simulink model "EM21"  (R2024a)
settings: Solver=VariableStepAuto  StartTime=0.0  StopTime=10.0  RelTol=1e-3
libraries: spsThreePhaseVIMeasurementLib x6, spsThreePhaseTransformerTwoWindingsLib x5, spsThreePhaseParallelRLCBranchLib x3, spsThreePhaseSourceLib x3, spsThreePhaseBreakerLib x3, sps_lib x1
settings Model: Creator=ASUS  LastModifiedBy=ASUS

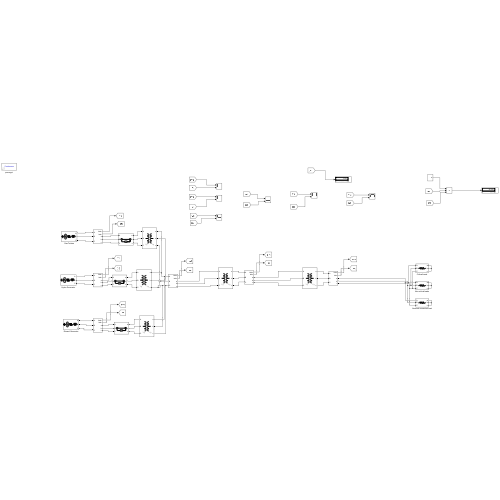
[thumbnail: Simulink's stored preview of the top-level diagram]
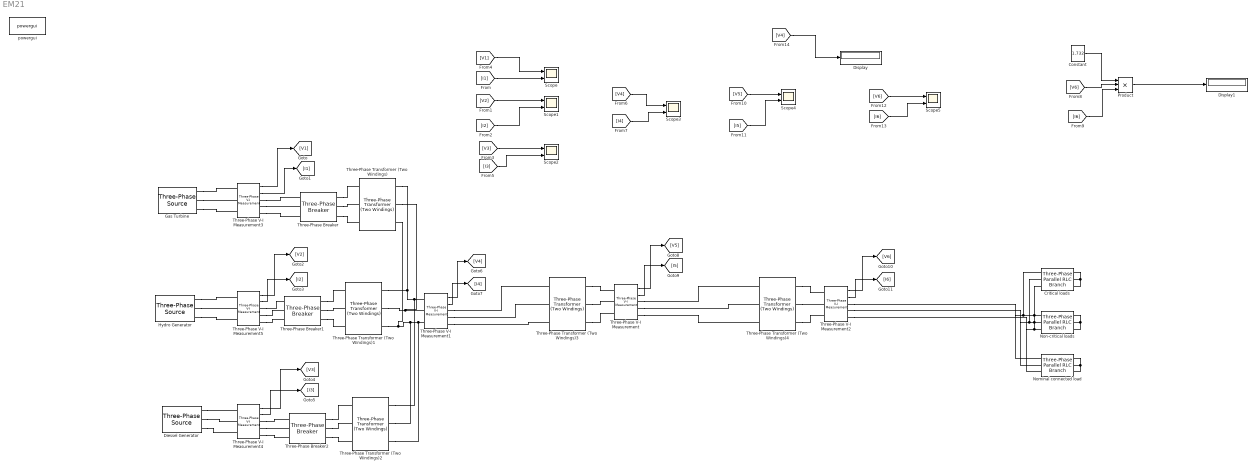
== system EM21 ==
  Constant : Constant  Value=1.732
  Critical loads : spsThreePhaseParallelRLCBranchLib/Three-Phase Parallel RLC Branch  LConnTagsString=A|B|C  RConnTagsString=A|B|C  BranchType=R  Resistance=1000  Inductance=1e-3  Capacitance=1e-6  Measurements=None
  Diessel Generator : spsThreePhaseSourceLib/Three-Phase Source  InternalConnection=Yg  VoltagePhases=off  Voltage=10e3  PhaseAngle=0  Voltage_phases=[25e3 25e3 25e3]/sqrt(3)  PhaseAngles_phases=[0 -120 +120]  Frequency=50  NonIdealSource=on  SpecifyImpedance=off  Resistance=0.8929  Inductance=16.58e-3  ShortCircuitLevel=100e6  BaseVoltage=10e3  XRratio=7  BusType=PV  Pref=4e6  Qref=0  Prefabc=[10e3, 10e3, 10e3]  Qrefabc=[0, 0, 0]  Qmin=-inf  Qmax=inf
  Display : Display
  Display1 : Display
  Gas Turbine : spsThreePhaseSourceLib/Three-Phase Source  InternalConnection=Yg  VoltagePhases=off  Voltage=11e3  PhaseAngle=0  Voltage_phases=[25e3 25e3 25e3]/sqrt(3)  PhaseAngles_phases=[0 -120 +120]  Frequency=50  NonIdealSource=on  SpecifyImpedance=off  Resistance=0.8929  Inductance=16.58e-3  ShortCircuitLevel=100e6  BaseVoltage=11e3  XRratio=7  BusType=PV  Pref=1e6  Qref=0  Prefabc=[10e3, 10e3, 10e3]  Qrefabc=[0, 0, 0]  Qmin=-inf  Qmax=inf
  Hydro Generator : spsThreePhaseSourceLib/Three-Phase Source  InternalConnection=Yg  VoltagePhases=off  Voltage=12e3  PhaseAngle=0  Voltage_phases=[25e3 25e3 25e3]/sqrt(3)  PhaseAngles_phases=[0 -120 +120]  Frequency=50  NonIdealSource=on  SpecifyImpedance=off  Resistance=0.8929  Inductance=16.58e-3  ShortCircuitLevel=100e6  BaseVoltage=12e3  XRratio=7  BusType=PV  Pref=2e6  Qref=0  Prefabc=[10e3, 10e3, 10e3]  Qrefabc=[0, 0, 0]  Qmin=-inf  Qmax=inf
  Nominal connected load : spsThreePhaseParallelRLCBranchLib/Three-Phase Parallel RLC Branch  LConnTagsString=A|B|C  RConnTagsString=A|B|C  BranchType=R  Resistance=1000  Inductance=1e-3  Capacitance=1e-6  Measurements=None
  Non-critical loads : spsThreePhaseParallelRLCBranchLib/Three-Phase Parallel RLC Branch  LConnTagsString=A|B|C  RConnTagsString=A|B|C  BranchType=R  Resistance=1000  Inductance=1e-3  Capacitance=1e-6  Measurements=None
  Product : Product  Inputs=3
  Scope{,1..5} (6 alike) : Scope  NumInputPorts=2
  Three-Phase Transformer (Two Windings) : spsThreePhaseTransformerTwoWindingsLib/Three-Phase Transformer (Two Windings)  Winding1Connection=Yg  Winding2Connection=Yg  CoreType=Three single-phase transformers  SetSaturation=off  Hysteresis=off  DataFile='hysteresis'  SetInitialFlux=off  Measurements=None  UNITS=pu  NominalPower=[ 1e6 , 50 ]  Winding1=[ 11e3 , 0.002 , 0.08 ]  Winding2=[ 132e3 , 0.002 , 0.08 ]  Rm=500  Lm=500  L0=2.866  Saturation=[ 0,0 ; 0.0024,1.2 ; 1.0,1.52 ]  InitialFluxes=[1273.5 -1273.5 1114.3]  BreakLoop=off  DiscreteSolver=Trapezoidal iterative  DataType=off  TransfoNumber=1
  Three-Phase Transformer (Two Windings)1 : spsThreePhaseTransformerTwoWindingsLib/Three-Phase Transformer (Two Windings)  Winding1Connection=Yg  Winding2Connection=Yg  CoreType=Three single-phase transformers  SetSaturation=off  Hysteresis=off  DataFile='hysteresis'  SetInitialFlux=off  Measurements=None  UNITS=pu  NominalPower=[ 2e6 , 50 ]  Winding1=[ 12e3 , 0.002 , 0.08 ]  Winding2=[ 132e3 , 0.002 , 0.08 ]  Rm=500  Lm=500  L0=0.5  Saturation=[ 0,0 ; 0.0024,1.2 ; 1.0,1.52 ]  InitialFluxes=[ 0.8 , -0.8 , 0.7 ]  BreakLoop=off  DiscreteSolver=Trapezoidal iterative  DataType=off  TransfoNumber=1
  Three-Phase Transformer (Two Windings)2 : spsThreePhaseTransformerTwoWindingsLib/Three-Phase Transformer (Two Windings)  Winding1Connection=Yg  Winding2Connection=Yg  CoreType=Three single-phase transformers  SetSaturation=off  Hysteresis=off  DataFile='hysteresis'  SetInitialFlux=off  Measurements=None  UNITS=pu  NominalPower=[ 4e6 , 50 ]  Winding1=[ 10e3 , 0.002 , 0.08 ]  Winding2=[ 132e3 , 0.002 , 0.08 ]  Rm=500  Lm=500  L0=0.5  Saturation=[ 0,0 ; 0.0024,1.2 ; 1.0,1.52 ]  InitialFluxes=[ 0.8 , -0.8 , 0.7 ]  BreakLoop=off  DiscreteSolver=Trapezoidal iterative  DataType=off  TransfoNumber=1
  Three-Phase Transformer (Two Windings)3 : spsThreePhaseTransformerTwoWindingsLib/Three-Phase Transformer (Two Windings)  Winding1Connection=Yg  Winding2Connection=Yg  CoreType=Three single-phase transformers  SetSaturation=off  Hysteresis=off  DataFile='hysteresis'  SetInitialFlux=off  Measurements=None  UNITS=pu  NominalPower=[ 7e6 , 50 ]  Winding1=[ 132e3 , 0.002 , 0.08 ]  Winding2=[ 11e3 , 0.002 , 0.08 ]  Rm=500  Lm=500  L0=0.5  Saturation=[ 0,0 ; 0.0024,1.2 ; 1.0,1.52 ]  InitialFluxes=[ 0.8 , -0.8 , 0.7 ]  BreakLoop=off  DiscreteSolver=Trapezoidal iterative  DataType=off  TransfoNumber=1
  Three-Phase Transformer (Two Windings)4 : spsThreePhaseTransformerTwoWindingsLib/Three-Phase Transformer (Two Windings)  Winding1Connection=Yg  Winding2Connection=Yg  CoreType=Three single-phase transformers  SetSaturation=off  Hysteresis=off  DataFile='hysteresis'  SetInitialFlux=off  Measurements=None  UNITS=pu  NominalPower=[ 7e6 , 50 ]  Winding1=[ 11e3 , 0.002 , 0.08 ]  Winding2=[ 400 , 0.002 , 0.08 ]  Rm=500  Lm=500  L0=0.5  Saturation=[ 0,0 ; 0.0024,1.2 ; 1.0,1.52 ]  InitialFluxes=[ 0.8 , -0.8 , 0.7 ]  BreakLoop=off  DiscreteSolver=Trapezoidal iterative  DataType=off  TransfoNumber=1
  Three-Phase V-I Measurement{,1..5} (6 alike) : spsThreePhaseVIMeasurementLib/Three-Phase V-I Measurement  VoltageMeasurement=phase-to-ground  SetLabelV=off  LabelV=Vabc  Vpu=off  VpuLL=off  CurrentMeasurement=yes  SetLabelI=off  LabelI=Iabc  Ipu=off  Pbase=100e6  Vbase=500e3  OutputType=Complex  PhasorSimulation=off  PSBequivalent=0
  Three-Phase Breaker : spsThreePhaseBreakerLib/Three-Phase Breaker  InitialState=closed  SwitchA=on  SwitchB=on  SwitchC=on  SwitchTimes="[1/60  5/60]"  External=off  BreakerResistance=0.01  SnubberResistance=1e6  SnubberCapacitance=inf  Measurements=None
  Three-Phase Breaker1 : spsThreePhaseBreakerLib/Three-Phase Breaker  InitialState=closed  SwitchA=on  SwitchB=on  SwitchC=on  SwitchTimes="[1/60  5/60]"  External=off  BreakerResistance=0.01  SnubberResistance=1e6  SnubberCapacitance=inf  Measurements=None
  Three-Phase Breaker2 : spsThreePhaseBreakerLib/Three-Phase Breaker  InitialState=closed  SwitchA=on  SwitchB=on  SwitchC=on  SwitchTimes="[1/60  5/60]"  External=off  BreakerResistance=0.01  SnubberResistance=1e6  SnubberCapacitance=inf  Measurements=None
  powergui : sps_lib/powergui  Priority=1  SimulationMode=Continuous  SampleTime=50e-6  frequency=60  Iterations=50  frequencyindice=50  Pbase=100e6  ErrMax=1e-4  UnitsV=kV  UnitsW=MW  buscounter=0  FunctionMessages=off  echomessages=off  EnableUseOfTLC=off  CurrentSourceSwitches=off  DisableSnubberDevices=off  DisableRonSwitches=off  DisableVfSwitches=off  DisplayEquations=off  AutomaticDiscreteSolvers=off  SolverType=Tustin/Backward Euler (TBE)  Interpol=off  ExternalGateDelay=off  methode=off  Ts=100  x0status=blocks  SPID=on  SwTol=0  HookPort=off  NonlinearTolerance=1e-4  nMaxIteration=100  ContinueOnMaxIteration=off  RestoreLinks=warning  ResistiveCurrentMeasurement=off  Frange=[0:2:500]  Ylog=off  Xlog=on  ShowGrid=off  save=off  variable=ZData  structure=0  ZoomFFT=off  StartTime=0.0  cycles=1  DisplayStyle=1  fundamental=60  FreqAxis=off  MaxFrequency=1000  frequencyindicesteady=1  RmsSteady=1  display=off
  wires:
  Three-Phase V-I Measurement3/1 -> [V1]
  Three-Phase V-I Measurement3/2 -> [I1]
  Three-Phase V-I Measurement5/1 -> [V2]
  Three-Phase V-I Measurement5/2 -> [I2]
  Three-Phase V-I Measurement4/1 -> [V3]
  Three-Phase V-I Measurement4/2 -> [I3]
  [V1] -> Scope/1
  [I1] -> Scope/2
  [V2] -> Scope1/1
  [I2] -> Scope1/2
  [V3] -> Scope2/1
  [I3] -> Scope2/2
  Three-Phase V-I Measurement1/1 -> [V4]
  Three-Phase V-I Measurement1/2 -> [I4]
  [V4] -> Scope3/1
  [I4] -> Scope3/2
  Three-Phase V-I Measurement/1 -> [V5]
  Three-Phase V-I Measurement/2 -> [I5]
  Three-Phase V-I Measurement2/1 -> [V6]
  Three-Phase V-I Measurement2/2 -> [I6]
  [V5] -> Scope4/1
  [I5] -> Scope4/2
  [V6] -> Scope5/1
  [I6] -> Scope5/2
  [V4] -> Display/1
  Constant/1 -> Product/1
  [V6] -> Product/2
  [I6] -> Product/3
  Product/1 -> Display1/1
  connections:
  Critical loads/RConn1 -- Critical loads/RConn2 -- Critical loads/RConn3
  Non-critical loads/RConn1 -- Non-critical loads/RConn2 -- Non-critical loads/RConn3
  Nominal connected load/RConn1 -- Nominal connected load/RConn2 -- Nominal connected load/RConn3
  Three-Phase Transformer (Two Windings)1/RConn1 -- Three-Phase Transformer (Two Windings)2/RConn1 -- Three-Phase V-I Measurement1/LConn1 -- Three-Phase Transformer (Two Windings)/RConn1
  Three-Phase Transformer (Two Windings)1/RConn2 -- Three-Phase Transformer (Two Windings)/RConn2 -- Three-Phase V-I Measurement1/LConn2
  Three-Phase Transformer (Two Windings)1/RConn3 -- Three-Phase Transformer (Two Windings)/RConn3 -- Three-Phase Transformer (Two Windings)2/RConn2 -- Three-Phase Transformer (Two Windings)2/RConn3 -- Three-Phase V-I Measurement1/LConn3
  Gas Turbine/RConn1 -- Three-Phase V-I Measurement3/LConn1
  Gas Turbine/RConn2 -- Three-Phase V-I Measurement3/LConn2
  Gas Turbine/RConn3 -- Three-Phase V-I Measurement3/LConn3
  Hydro Generator/RConn1 -- Three-Phase V-I Measurement5/LConn1
  Hydro Generator/RConn2 -- Three-Phase V-I Measurement5/LConn2
  Hydro Generator/RConn3 -- Three-Phase V-I Measurement5/LConn3
  Diessel Generator/RConn1 -- Three-Phase V-I Measurement4/LConn1
  Diessel Generator/RConn2 -- Three-Phase V-I Measurement4/LConn2
  Diessel Generator/RConn3 -- Three-Phase V-I Measurement4/LConn3
  Three-Phase V-I Measurement3/RConn1 -- Three-Phase Breaker/LConn1
  Three-Phase V-I Measurement3/RConn2 -- Three-Phase Breaker/LConn2
  Three-Phase V-I Measurement3/RConn3 -- Three-Phase Breaker/LConn3
  Three-Phase V-I Measurement5/RConn1 -- Three-Phase Breaker1/LConn1
  Three-Phase V-I Measurement5/RConn2 -- Three-Phase Breaker1/LConn2
  Three-Phase V-I Measurement5/RConn3 -- Three-Phase Breaker1/LConn3
  Three-Phase V-I Measurement4/RConn1 -- Three-Phase Breaker2/LConn1
  Three-Phase V-I Measurement4/RConn2 -- Three-Phase Breaker2/LConn2
  Three-Phase V-I Measurement4/RConn3 -- Three-Phase Breaker2/LConn3
  Three-Phase Breaker/RConn1 -- Three-Phase Transformer (Two Windings)/LConn1
  Three-Phase Breaker/RConn2 -- Three-Phase Transformer (Two Windings)/LConn2
  Three-Phase Breaker/RConn3 -- Three-Phase Transformer (Two Windings)/LConn3
  Three-Phase Breaker1/RConn1 -- Three-Phase Transformer (Two Windings)1/LConn1
  Three-Phase Breaker1/RConn2 -- Three-Phase Transformer (Two Windings)1/LConn2
  Three-Phase Breaker1/RConn3 -- Three-Phase Transformer (Two Windings)1/LConn3
  Three-Phase Breaker2/RConn1 -- Three-Phase Transformer (Two Windings)2/LConn1
  Three-Phase Breaker2/RConn2 -- Three-Phase Transformer (Two Windings)2/LConn2
  Three-Phase Breaker2/RConn3 -- Three-Phase Transformer (Two Windings)2/LConn3
  Non-critical loads/LConn1 -- Three-Phase V-I Measurement2/RConn1 -- Nominal connected load/LConn1 -- Critical loads/LConn1
  Non-critical loads/LConn2 -- Nominal connected load/LConn2 -- Three-Phase V-I Measurement2/RConn2 -- Critical loads/LConn2
  Non-critical loads/LConn3 -- Nominal connected load/LConn3 -- Three-Phase V-I Measurement2/RConn3 -- Critical loads/LConn3
  Three-Phase V-I Measurement1/RConn1 -- Three-Phase Transformer (Two Windings)3/LConn1
  Three-Phase V-I Measurement1/RConn2 -- Three-Phase Transformer (Two Windings)3/LConn2
  Three-Phase V-I Measurement1/RConn3 -- Three-Phase Transformer (Two Windings)3/LConn3
  Three-Phase Transformer (Two Windings)3/RConn1 -- Three-Phase V-I Measurement/LConn1
  Three-Phase Transformer (Two Windings)3/RConn2 -- Three-Phase V-I Measurement/LConn2
  Three-Phase Transformer (Two Windings)3/RConn3 -- Three-Phase V-I Measurement/LConn3
  Three-Phase V-I Measurement/RConn1 -- Three-Phase Transformer (Two Windings)4/LConn1
  Three-Phase V-I Measurement/RConn2 -- Three-Phase Transformer (Two Windings)4/LConn2
  Three-Phase V-I Measurement/RConn3 -- Three-Phase Transformer (Two Windings)4/LConn3
  Three-Phase Transformer (Two Windings)4/RConn1 -- Three-Phase V-I Measurement2/LConn1
  Three-Phase Transformer (Two Windings)4/RConn2 -- Three-Phase V-I Measurement2/LConn2
  Three-Phase Transformer (Two Windings)4/RConn3 -- Three-Phase V-I Measurement2/LConn3
